simulink model "Malha_Fechada_2016"  (R2021a)
settings: Solver=VariableStepAuto  StartTime=0.0  StopTime=10.0  RelTol=1e-3
values from neighbouring files (symbols this model uses):
  Cd = c2d(C,T,'matched')    [Efeitos_MF.m]
  f = 1/T    (= 5)    [Efeitos_MF.m]
settings Model: Creator=ribei  LastModifiedBy=check
settings SolverCC: AlgebraicLoopSolver=TrustRegion
settings DebuggingCC: UnconnectedInputMsg=none  UnconnectedOutputMsg=none  UnconnectedLineMsg=none  SFMachineParentedDataDiag=warning  ArithmeticOperatorsInVariantConditions=warning
settings ModelReferenceCC: EnableRefExpFcnMdlSchedulingChecks=off
settings SFSimCC: CustomCodeUndefinedFunction=UseInterfaceOnly
settings RTWCC: Description=Generic Real-Time Target
settings CodeAppCC: StateflowObjectComments=on

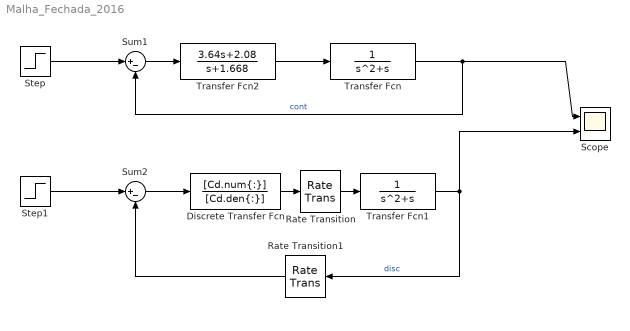
== system Malha_Fechada_2016 ==
  Discrete Transfer Fcn : DiscreteTransferFcn  Numerator=[Cd.num{:}]  Denominator=[Cd.den{:}]
  Rate Transition : RateTransition  Integrity=off  OutPortSampleTimeOpt=Inherit
  Rate Transition1 : RateTransition  OutPortSampleTime=1/f
  Scope : Scope  NumInputPorts=2
  Step : Step  SampleTime=0
  Step1 : Step  SampleTime=1/f
  Sum1 : Sum  Inputs=|+-
  Sum2 : Sum  Inputs=|+-
  Transfer Fcn : TransferFcn  Denominator=[1 1 0]
  Transfer Fcn1 : TransferFcn  Denominator=[1 1 0]
  Transfer Fcn2 : TransferFcn  Numerator=[3.64 2.08]  Denominator=[1 1.668]
  wires:
  Sum1/1 -> Transfer Fcn2/1
  Step/1 -> Sum1/1
  Transfer Fcn/1 -> Sum1/2, Scope/1  "cont"
  Transfer Fcn2/1 -> Transfer Fcn/1
  Discrete Transfer Fcn/1 -> Rate Transition/1
  Sum2/1 -> Discrete Transfer Fcn/1
  Rate Transition1/1 -> Sum2/2
  Step1/1 -> Sum2/1
  Rate Transition/1 -> Transfer Fcn1/1
  Transfer Fcn1/1 -> Rate Transition1/1, Scope/2  "disc"
